simulink model "Lab2_ADC_modeling_SAR"  (R2023b)
settings: Solver=VariableStepAuto  StartTime=0.0  StopTime=N*Ts  RelTol=1e-3
values from neighbouring files (symbols this model uses):
  ampl = 0.45    [Lab1.m]    (also in Lab2.m; Question_4_Differential.m)
  N = 4096    [Lab1.m]    (also in Lab2.m; Question_4_Differential.m)
  offset = 0.5    [Lab1.m]    (also in Lab2.m; Question_4_Differential.m)
  Ts = 1/fs    (= 1e-08)    [Lab1.m]    (also in Lab2.m; Question_4_Differential.m)
libraries: simulink_extras x1, simulink x1, dspsigops x1
settings Model: Creator=gerardo.salgado  LastModifiedBy=mofa
settings SolverCC: AlgebraicLoopSolver=TrustRegion
settings DataIOCC: ReturnWorkspaceOutputs=off
settings DebuggingCC: ArithmeticOperatorsInVariantConditions=warning
settings ModelReferenceCC: EnableRefExpFcnMdlSchedulingChecks=on
settings SFSimCC: SimUseLocalCustomCode=off  CustomCodeUndefinedFunction=UseInterfaceOnly
settings RTWCC: RTWUseLocalCustomCode=off
settings CodeAppCC: StateflowObjectComments=on

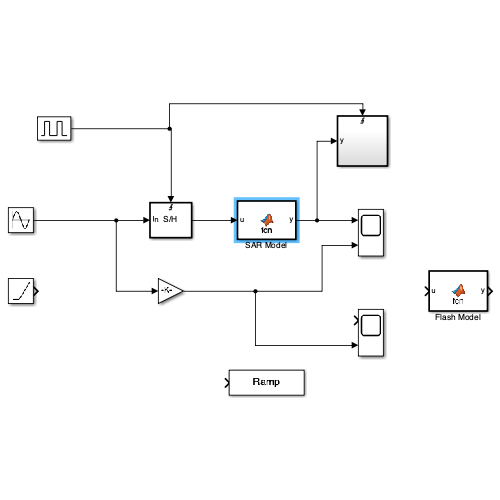
[thumbnail: Simulink's stored preview of the top-level diagram]
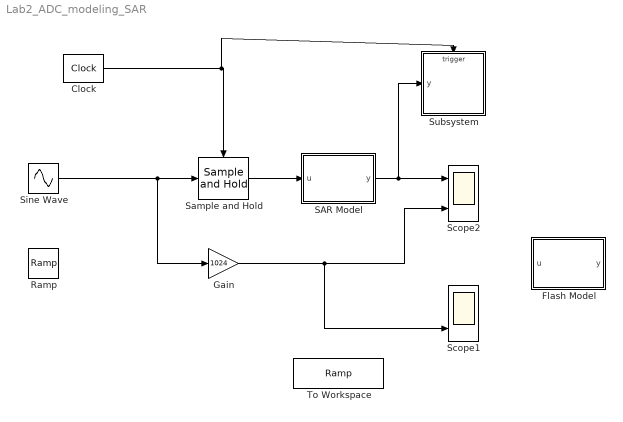
== system Lab2_ADC_modeling_SAR ==
  Clock : simulink_extras/Flip Flops/Clock  period=Ts
  Flash Model : MATLAB Function  TreatAsAtomicUnit=on
  Gain : Gain  Gain=1024
  Ramp : simulink/Sources/Ramp  slope=1/(N*Ts)  start=0  InitialOutput=0
  SAR Model : MATLAB Function  TreatAsAtomicUnit=on
  Sample and Hold : dspsigops/Sample and Hold  trig=Rising edge  initCond=0  latchinput=off
  Scope1 : Scope  NumInputPorts=2
  Scope2 : Scope  NumInputPorts=2
  Sine Wave : Sin  Amplitude=ampl  Bias=offset  Frequency=2*pi*fi  SampleTime=0
  Subsystem : Subsystem
  To Workspace : ToWorkspace  VariableName=Ramp  SampleTime=-1
      settings: Save2DSignal=2-D array (concatenate along first dimension)
  wires:
  Clock/1 -> Subsystem/Trigger, Sample and Hold/Trigger
  SAR Model/1(y) -> Subsystem/1(y), Scope2/1
  Sample and Hold/1 -> SAR Model/1(u)
  Gain/1 -> Scope2/2, Scope1/2
  Sine Wave/1 -> Gain/1, Sample and Hold/1

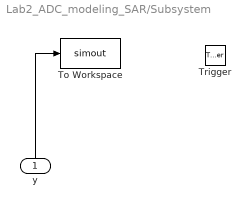
== system Lab2_ADC_modeling_SAR/Subsystem ==
  y : Inport
  Trigger : TriggerPort  VariantControl=Variant  PortDimensions=1
  To Workspace : ToWorkspace  VariableName=simout  SampleTime=-1
      settings: Save2DSignal=2-D array (concatenate along first dimension)
  wires:
  y/1 -> To Workspace/1

== matlab function Lab2_ADC_modeling_SAR/Flash Model ==
  data: u input; y output
function y = fcn(u)
vin=u;

Nbit=10;                        %%Number of bits.

LSB=1/2^Nbit;                   %%LSB size (considers Vp=1 and Vn=0).
rladder=[1:1:2^Nbit-1]*LSB;     %%%Reference voltage generation.
vout=ones(1,2^Nbit-1);          %%%Formal initialisation of vout variable.  

p=0.0/100;                      %%percentage of mismatch
randn('seed', 31233);           %% Uses a fixed seed for the PRNG
mismatch=randn(1,2^Nbit-1)*p;   %%Random variable to be added to rladder
rladder=rladder.*(1+mismatch);  %%Mismatch added to rladder.

for i=1:1:2^Nbit-1              %%2^Nbit -1 comparators 
    if vin<rladder(i)           %%Vin Compared agains the different voltages
                                %%In the rladder
        vout(i)=0;              %%Output is 0 if the vin is < a given rladder
    else 
        vout(i)=1;              %%Output is 1 if vin is larger.
    end
end

y=sum(vout);

== matlab function Lab2_ADC_modeling_SAR/SAR Model ==
  data: u input; y output
function y = fcn(u)
vin=u;

Nbit=10;                    %%%Number of bits 

Vcdac = 1./2.^[1:1:Nbit];   %%Voltage vector from CDAC.
 
vx = -vin;                  %%%Models bottom plate sampling

sar=ones(1,Nbit);           %%%Fromal initialization of variable

% PART (i) Capacitor mismatch
cap_p = 0.0/100;
% randn('seed', 31233);
randn('seed', 31233);
mismatch = randn(1,Nbit)*cap_p;

Vcdac = Vcdac.*(1+mismatch);

comp_p = 0.0/100;
comparator_mismatch = randn(1,Nbit)*comp_p;



for i=1:1:Nbit

    vx=vx+Vcdac(i);         %%%Bit Trial
    
        if vx > 0;          %%%Comparator Model  
            sar(i)=0;       %%%i-th digital output
                vx=vx-Vcdac(i); %%%Bit trial goes low
        else
            sar(i)=1;       %%%i-th digital output
                vx=vx;      %%%Bit trial remains high
    end
end

weights=2.^[0:1:Nbit-1];
weights=fliplr(weights);
y=sum(sar.*weights);
